simulink model "ep_5_4_4"  (R2023b)
settings: Solver=VariableStepAuto  StartTime=0.0  StopTime=10.0  RelTol=1e-3
settings Model: Creator=86186  LastModifiedBy=86186

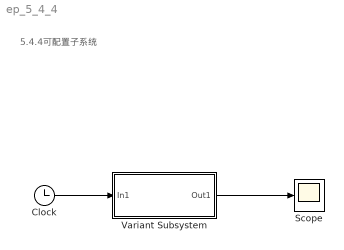
== system ep_5_4_4 ==
  note: 5.4.4可配置子系统
  Clock : Clock
  Scope : Scope
  Variant Subsystem : Subsystem  Variant=on  VariantControlMode=label  LabelModeActiveChoice=Subsystem2
  wires:
  Clock/1 -> Variant Subsystem/1(In1)
  Variant Subsystem/1(Out1) -> Scope/1

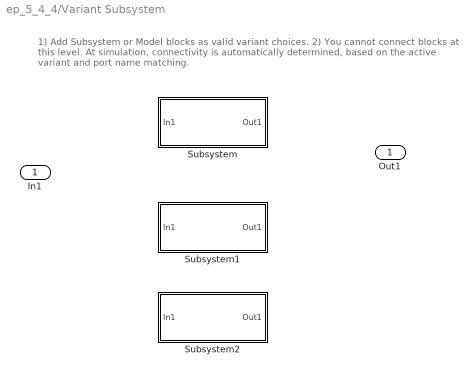
== system ep_5_4_4/Variant Subsystem ==
  note: 1) Add Subsystem or Model blocks as valid variant choices.
      | 2) You cannot connect blocks at this level. At simulation, connectivity is automatically
      | determined, based on the active variant and port name matching.
  In1 : Inport
  Subsystem : Subsystem  VariantControl=Subsystem
  Subsystem1 : Subsystem  VariantControl=Subsystem1
  Subsystem2 : Subsystem  VariantControl=Subsystem2
  Out1 : Outport

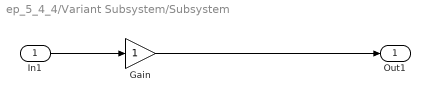
== system ep_5_4_4/Variant Subsystem/Subsystem ==
  In1 : Inport
  Gain : Gain
  Out1 : Outport
  wires:
  Gain/1 -> Out1/1
  In1/1 -> Gain/1

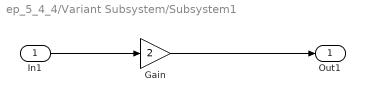
== system ep_5_4_4/Variant Subsystem/Subsystem1 ==
  In1 : Inport
  Gain : Gain  Gain=2
  Out1 : Outport
  wires:
  In1/1 -> Gain/1
  Gain/1 -> Out1/1

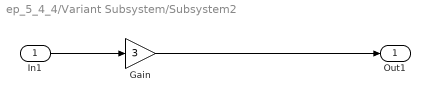
== system ep_5_4_4/Variant Subsystem/Subsystem2 ==
  In1 : Inport
  Gain : Gain  Gain=3
  Out1 : Outport
  wires:
  In1/1 -> Gain/1
  Gain/1 -> Out1/1
